simulink model "trajectory_planner"  (R2014b)
settings: Solver=ode45  SolverMode=SingleTasking  StartTime=0.0  StopTime=simtime  RelTol=1e-3
values from neighbouring files (symbols this model uses):
  amax = 255    [workshopB.m]
  amin = -amax    (= -255)    [workshopB.m]
  F_c = 1.5e-3    (= 0.0015)    [workshopB.m]
  J1 = 0.0006    [workshopB.m]
  motor = motor_pars    [workshopB.m]
  n = 5    [workshopB.m]
  t1 = sqrt(rs/amax)    [workshopB.m]
  t2 = t1    [workshopB.m]
  t3 = t1+t2    [workshopB.m]
  Ts = 0.01    [workshopB.m]
libraries: simulink x3
settings Model: Creator=Gabriel  LastModifiedBy=es2lab2
settings SolverCC: ZeroCrossAlgorithm=Adaptive
settings OptimizationCC: BlockReduction=off  BooleanDataType=off  UseDivisionForNetSlopeComputation=off  SimCompilerOptimization=off
settings DebuggingCC: SaveWithParameterizedLinksMsg=none  UnderspecifiedInitializationDetection=Classic  MergeDetectMultiDrivingBlocksExec=none  SignalResolutionControl=TryResolveAllWithWarning  SolverPrmCheckMsg=none  FrameProcessingCompatibilityMsg=error  AllowSymbolicDim=off
settings HardwareCC: TargetUnknown=on
settings RTWCC: RTWCompilerOptimization=off
settings ConfigComp: CovMetricSettings=dw  CovHtmlReporting=on  CovSaveCumulativeToWorkspaceVar=on  CovSaveSingleToWorkspaceVar=on  CovModelRefEnable=Off  CovExternalEMLEnable=off  CovSFcnEnable=off

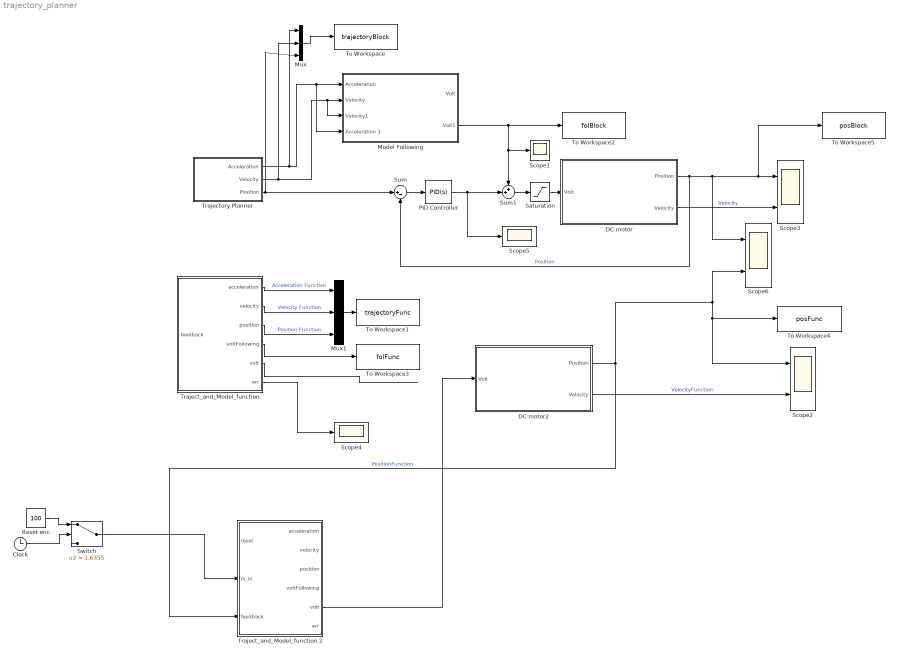
== system trajectory_planner ==
  Clock : Clock
  DC motor : Subsystem
  DC motor2 : Subsystem
  Model Following : Subsystem
  Mux : Mux  Inputs=3
  Mux1 : Mux  Inputs=3
  PID Controller : simulink/Continuous/PID Controller  Controller=PID  TimeDomain=Continuous-time  SampleTime=-1  IntegratorMethod=Forward Euler  FilterMethod=Forward Euler  Form=Parallel  P=1  I=1  D=0  N=100  InitialConditionSource=internal  InitialConditionForIntegrator=0  InitialConditionForFilter=0  ExternalReset=none  LimitOutput=off  UpperSaturationLimit=inf  LowerSaturationLimit=-inf  LinearizeAsGain=on  AntiWindupMode=none  Kb=1  TrackingMode=off  Kt=1  PParamMin=[]  PParamMax=[]  IParamMin=[]  IParamMax=[]  DParamMin=[]  DParamMax=[]  NParamMin=[]  NParamMax=[]  KbParamMin=[]  KbParamMax=[]  KtParamMin=[]  KtParamMax=[]  POutMin=[]  POutMax=[]  IOutMin=[]  IOutMax=[]  DOutMin=[]  DOutMax=[]  NOutMin=[]  NOutMax=[]  KbOutMin=[]  KbOutMax=[]  KtOutMin=[]  KtOutMax=[]  IntegratorOutMin=[]  IntegratorOutMax=[]  FilterOutMin=[]  FilterOutMax=[]  SumOutMin=[]  SumOutMax=[]  SumI1OutMin=[]  SumI1OutMax=[]  SumI2OutMin=[]  SumI2OutMax=[]  SumI3OutMin=[]  SumI3OutMax=[]  SumDOutMin=[]  SumDOutMax=[]  SaturationOutMin=[]  SaturationOutMax=[]  IntegratorContinuousStateAttributes=''  IntegratorStateMustResolveToSignalObject=off  IntegratorRTWStateStorageClass=Auto  FilterContinuousStateAttributes=''  FilterStateMustResolveToSignalObject=off  FilterRTWStateStorageClass=Auto  DifferentiatorICPrevScaledInput=0  DifferentiatorOutMin=[]  DifferentiatorOutMax=[]  UseFilter=on
  Reset enc : Constant  Value=100
  Saturation : Saturate  UpperLimit=24  LowerLimit=-24
  Scope1 : Scope
      settings: TimeRange=7.551351351351352  YMin=-14.3868  YMax=28.08299  SaveName=ScopeData2
  Scope2 : Scope  NumInputPorts=2
      settings: ShowLegends=on  TimeRange=7.551351351351352  YMin=-6.917~-5  YMax=57.3125~5
  Scope3 : Scope  NumInputPorts=2
      settings: ShowLegends=on  TimeRange=7.551351351351352  YMin=-19.9609  YMax=179.64809  SaveName=ScopeData5
  Scope4 : Scope
      settings: TimeRange=7.551351351351352  YMin=-110.7141  YMax=44.80519
  Scope5 : Scope
      settings: TimeRange=7.551351351351352  YMin=-0.000000000000008  YMax=0.000000000000029  SaveName=ScopeData8
  Scope6 : Scope  NumInputPorts=2
      settings: ShowLegends=on  TimeRange=7.551351351351352  YMin=-12.6475~-5  YMax=113.827~5  SaveName=ScopeData3
  Sum : Sum  Inputs=|+-
  Sum1 : Sum  Inputs=++|
  Switch : Switch  Criteria=u2 > Threshold  Threshold=1.6355
  To Workspace : ToWorkspace  VariableName=trajectoryBlock  SaveFormat=Timeseries  SampleTime=-1
  To Workspace1 : ToWorkspace  VariableName=trajectoryFunc  SaveFormat=Timeseries  SampleTime=-1
  To Workspace2 : ToWorkspace  VariableName=folBlock  SaveFormat=Timeseries  SampleTime=-1
  To Workspace3 : ToWorkspace  VariableName=folFunc  SaveFormat=Timeseries  SampleTime=-1
  To Workspace4 : ToWorkspace  VariableName=posFunc  SaveFormat=Timeseries  SampleTime=-1
  To Workspace5 : ToWorkspace  VariableName=posBlock  SaveFormat=Timeseries  SampleTime=-1
  "Traject_and_Model_function " : MATLAB Function  TreatAsAtomicUnit=on  SystemSampleTime=Ts
  Traject_and_Model_function 2 : MATLAB Function  TreatAsAtomicUnit=on  SystemSampleTime=Ts
  Trajectory Planner : Subsystem
  wires:
  Sum/1 -> PID Controller/1
  DC motor/1(Position) -> Sum/2, Scope6/1, To Workspace5/1, Scope3/1  "Position"
  PID Controller/1 -> Sum1/2, Scope5/1
  Trajectory Planner/3(Position) -> Sum/1, Mux/3
  Trajectory Planner/1(Acceleration) -> Mux/1, Model Following/4(Acceleration 1), Model Following/1("Acceleration ")
  Trajectory Planner/2(Velocity) -> Model Following/3(Velocity1), Model Following/2(Velocity), Mux/2
  DC motor/2(Velocity) -> Scope3/2  "Velocity"
  Sum1/1 -> Saturation/1
  Saturation/1 -> DC motor/1(Volt)
  "Traject_and_Model_function "/5(volt) -> ?
  DC motor2/1(Position) -> Traject_and_Model_function 2/3(feedback), Scope6/2, Scope2/1, To Workspace4/1  "PositionFunction"
  DC motor2/2(Velocity) -> Scope2/2  "VelocityFunction"
  Model Following/2(Volt1) -> Sum1/1, Scope1/1, To Workspace2/1
  "Traject_and_Model_function "/1(acceleration) -> Mux1/1  "Acceleration Function"
  "Traject_and_Model_function "/2(velocity) -> Mux1/2  "Velocity Function"
  "Traject_and_Model_function "/3(position) -> Mux1/3  "Position Function"
  Mux/1 -> To Workspace/1
  Mux1/1 -> To Workspace1/1
  "Traject_and_Model_function "/4(voltFollowing) -> To Workspace3/1
  "Traject_and_Model_function "/6(err) -> Scope4/1
  Traject_and_Model_function 2/5(volt) -> DC motor2/1(Volt)
  Reset enc/1 -> Switch/1
  Clock/1 -> Switch/2
  Switch/1 -> Traject_and_Model_function 2/2(rs_in)

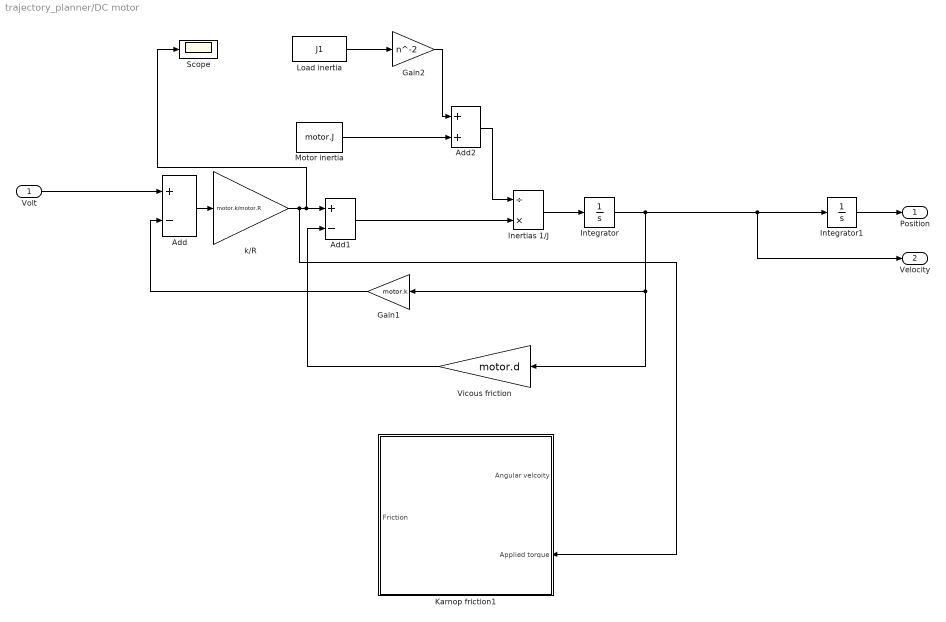
== system trajectory_planner/DC motor ==
  Volt : Inport
  Add : Sum  Inputs=+-
  Add1 : Sum  Inputs=+-
  Add2 : Sum
  Gain1 : Gain  Gain=motor.k
  Gain2 : Gain  Gain=n^-2
  Inertias 1/J : Product  Inputs=/*
  Integrator : Integrator
  Integrator1 : Integrator
  Karnop friction1 : Subsystem
  Load inertia : Constant  Value=J1
  Motor inertia : Constant  Value=motor.J
  Scope : Scope
  Vicous friction : Gain  Gain=motor.d
  "k/R " : Gain  Gain=motor.k/motor.R
  Position : Outport
  Velocity : Outport  Port=2
  wires:
  Vicous friction/1 -> Add1/2
  Add2/1 -> Inertias 1/J/1
  Gain2/1 -> Add2/1
  Load inertia/1 -> Gain2/1
  Motor inertia/1 -> Add2/2
  Integrator/1 -> Integrator1/1, Velocity/1, Vicous friction/1, Gain1/1
  Volt/1 -> Add/1
  Add1/1 -> Inertias 1/J/2
  Integrator1/1 -> Position/1
  Inertias 1/J/1 -> Integrator/1
  "k/R "/1 -> Scope/1, Add1/1, Karnop friction1/2(Applied torque)
  Add/1 -> "k/R "/1
  Gain1/1 -> Add/2

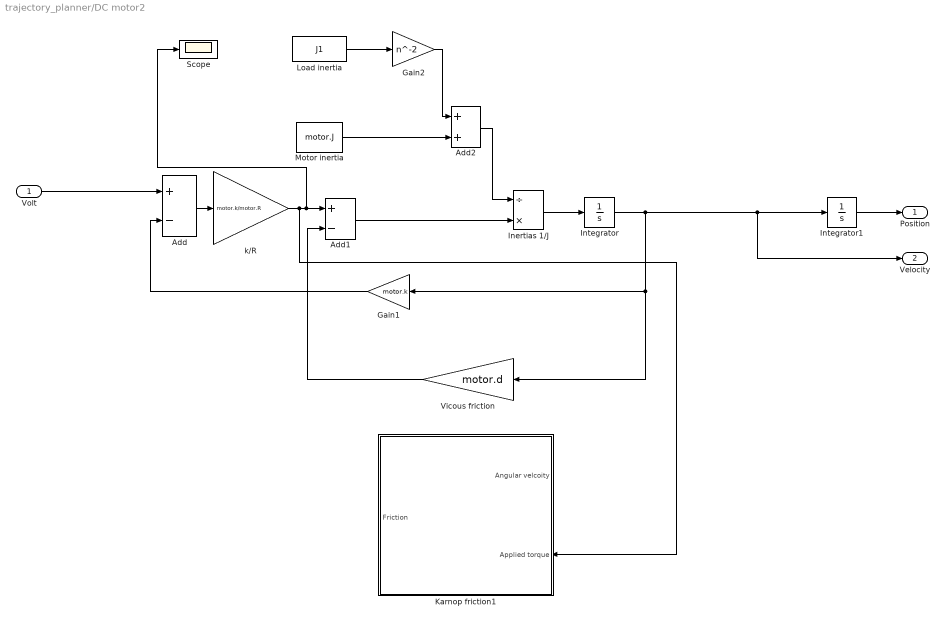
== system trajectory_planner/DC motor2 ==
  Volt : Inport
  Add : Sum  Inputs=+-
  Add1 : Sum  Inputs=+-
  Add2 : Sum
  Gain1 : Gain  Gain=motor.k
  Gain2 : Gain  Gain=n^-2
  Inertias 1/J : Product  Inputs=/*
  Integrator : Integrator
  Integrator1 : Integrator
  Karnop friction1 : Subsystem
  Load inertia : Constant  Value=J1
  Motor inertia : Constant  Value=motor.J
  Scope : Scope
  Vicous friction : Gain  Gain=motor.d
  "k/R " : Gain  Gain=motor.k/motor.R
  Position : Outport
  Velocity : Outport  Port=2
  wires:
  Gain1/1 -> Add/2
  Add/1 -> "k/R "/1
  "k/R "/1 -> Karnop friction1/2(Applied torque), Add1/1, Scope/1
  Inertias 1/J/1 -> Integrator/1
  Integrator1/1 -> Position/1
  Add1/1 -> Inertias 1/J/2
  Volt/1 -> Add/1
  Integrator/1 -> Vicous friction/1, Gain1/1, Velocity/1, Integrator1/1
  Motor inertia/1 -> Add2/2
  Load inertia/1 -> Gain2/1
  Gain2/1 -> Add2/1
  Add2/1 -> Inertias 1/J/1
  Vicous friction/1 -> Add1/2

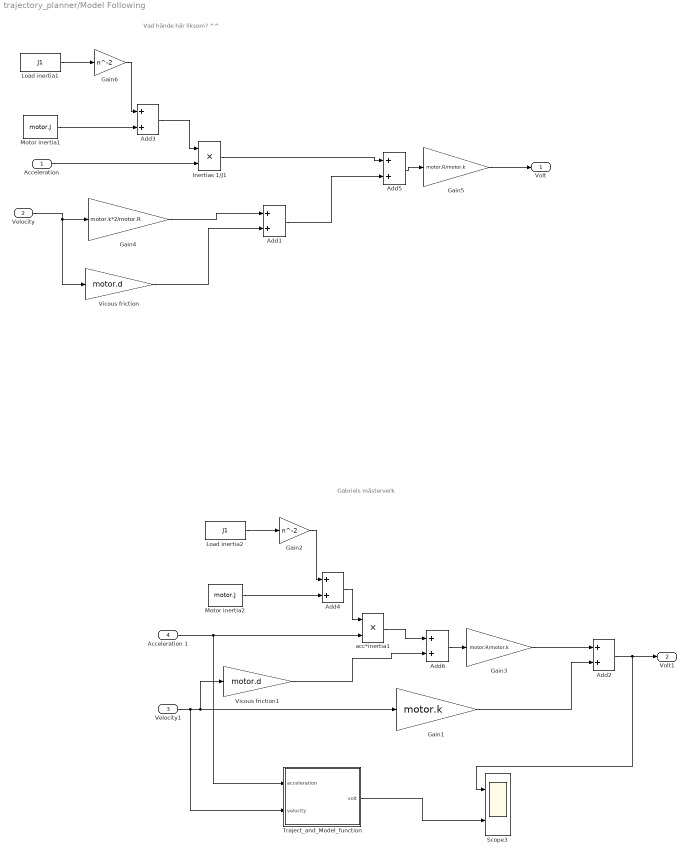
== system trajectory_planner/Model Following ==
  note: Vad hände här liksom? ^^
  note: Gabriels mästerverk
  "Acceleration " : Inport
  Velocity : Inport  Port=2
  Velocity1 : Inport  Port=3
  Acceleration 1 : Inport  Port=4
  Add{1..6} (6 alike) : Sum
  Gain1 : Gain  Gain=motor.k
  Gain2 : Gain  Gain=n^-2
  Gain3 : Gain  Gain=motor.R/motor.k
  Gain4 : Gain  Gain=motor.k*2/motor.R
  Gain5 : Gain  Gain=motor.R/motor.k
  Gain6 : Gain  Gain=n^-2
  Inertias 1/J1 : Product  Inputs=**
  Load inertia1 : Constant  Value=J1
  Load inertia2 : Constant  Value=J1
  Motor inertia1 : Constant  Value=motor.J
  Motor inertia2 : Constant  Value=motor.J
  Scope3 : Scope  NumInputPorts=2
      settings: ShowLegends=on  TimeRange=7.551351351351352  YMin=-14.3868  YMax=28.08299  SaveName=ScopeData4
  "Traject_and_Model_function " : MATLAB Function  TreatAsAtomicUnit=on  SystemSampleTime=Ts
  Vicous friction : Gain  Gain=motor.d
  Vicous friction1 : Gain  Gain=motor.d
  acc*inertia1 : Product  Inputs=**
  Volt : Outport
  Volt1 : Outport  Port=2
  wires:
  "Acceleration "/1 -> Inertias 1/J1/2
  Velocity/1 -> Vicous friction/1, Gain4/1
  Add3/1 -> Inertias 1/J1/1
  Gain6/1 -> Add3/1
  Load inertia1/1 -> Gain6/1
  Motor inertia1/1 -> Add3/2
  Vicous friction/1 -> Add1/2
  Gain5/1 -> Volt/1
  Add5/1 -> Gain5/1
  Inertias 1/J1/1 -> Add5/1
  Gain4/1 -> Add1/1
  Add1/1 -> Add5/2
  Velocity1/1 -> "Traject_and_Model_function "/2(velocity), Gain1/1, Vicous friction1/1
  Gain1/1 -> Add2/2
  Acceleration 1/1 -> "Traject_and_Model_function "/1(acceleration), acc*inertia1/2
  Add4/1 -> acc*inertia1/1
  Gain2/1 -> Add4/1
  Load inertia2/1 -> Gain2/1
  Motor inertia2/1 -> Add4/2
  Vicous friction1/1 -> Add6/2
  acc*inertia1/1 -> Add6/1
  Add6/1 -> Gain3/1
  Gain3/1 -> Add2/1
  Add2/1 -> Scope3/1, Volt1/1
  "Traject_and_Model_function "/1(volt) -> Scope3/2

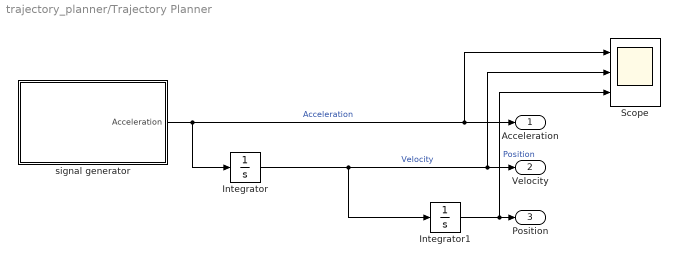
== system trajectory_planner/Trajectory Planner ==
  Integrator : Integrator
  Integrator1 : Integrator
  Scope : Scope  NumInputPorts=3
      settings: ShowLegends=on  YMin=-318.75~-5~-5  YMax=318.75~5~5
  signal generator : Subsystem
  Acceleration : Outport
  Velocity : Outport  Port=2
  Position : Outport  Port=3
  wires:
  signal generator/1(Acceleration) -> Integrator/1, Scope/1, Acceleration/1  "Acceleration"
  Integrator/1 -> Scope/2, Velocity/1, Integrator1/1  "Velocity"
  Integrator1/1 -> Scope/3, Position/1  "Position"

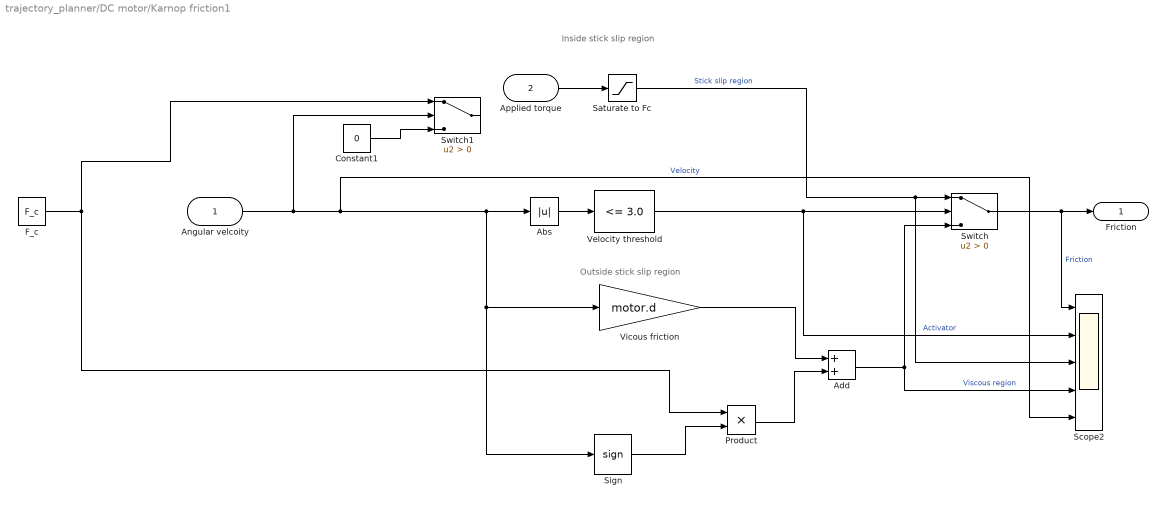
== system trajectory_planner/DC motor/Karnop friction1 ==
  note: Outside stick slip region
  note: Inside stick slip region
  Angular velcoity : Inport
  Applied torque : Inport  Port=2
  Abs : Abs  ZeroCross=off
  Add : Sum
  Constant1 : Constant  Value=0
  F_c : Constant  Value=F_c
  Product : Product
  Saturate to Fc : Saturate  UpperLimit=F_c  LowerLimit=-F_c  ZeroCross=off
  Scope2 : Scope  NumInputPorts=5
  Sign : Signum  ZeroCross=off
  Switch : Switch  Criteria=u2 > Threshold  ZeroCross=off
  Switch1 : Switch  Criteria=u2 > Threshold  ZeroCross=off
  "Velocity threshold " : simulink/Logic and Bit Operations/Compare To Constant  relop=<=  const=3.0  OutDataTypeStr=boolean
  Vicous friction : Gain  Gain=motor.d
  Friction : Outport
  wires:
  Applied torque/1 -> Saturate to Fc/1
  Add/1 -> Scope2/4, Switch/3  "Viscous region"
  Sign/1 -> Product/2
  F_c/1 -> Product/1, Switch1/1
  Vicous friction/1 -> Add/1
  Product/1 -> Add/2
  Abs/1 -> "Velocity threshold "/1
  "Velocity threshold "/1 -> Switch/2, Scope2/2  "Activator"
  Angular velcoity/1 -> Switch1/2, Sign/1, Vicous friction/1, Abs/1, Scope2/5  "Velocity"
  Switch/1 -> Friction/1, Scope2/1  "Friction"
  Saturate to Fc/1 -> Switch/1, Scope2/3  "Stick slip region"
  Constant1/1 -> Switch1/3

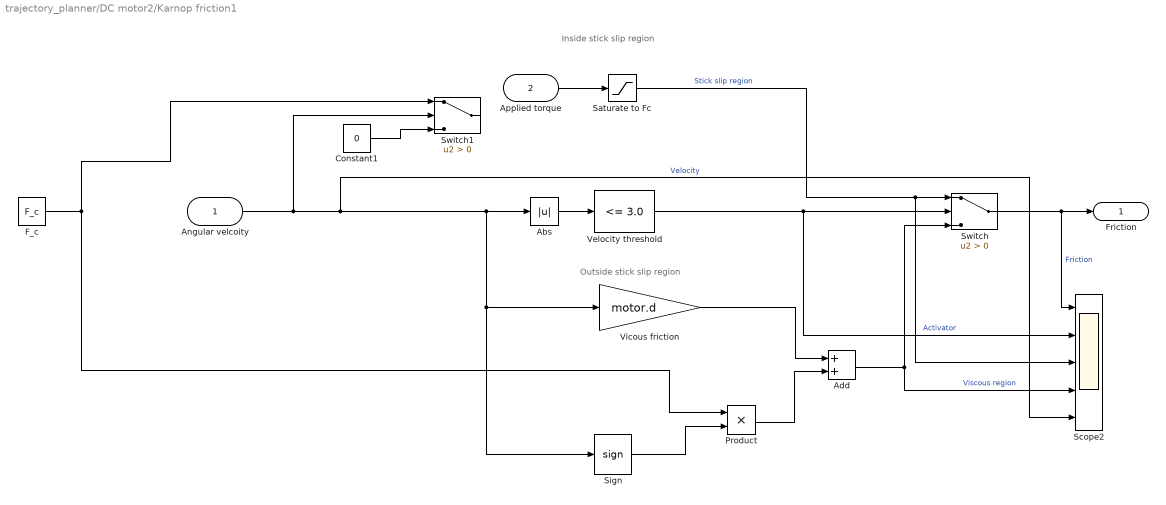
== system trajectory_planner/DC motor2/Karnop friction1 ==
  note: Inside stick slip region
  note: Outside stick slip region
  Angular velcoity : Inport
  Applied torque : Inport  Port=2
  Abs : Abs  ZeroCross=off
  Add : Sum
  Constant1 : Constant  Value=0
  F_c : Constant  Value=F_c
  Product : Product
  Saturate to Fc : Saturate  UpperLimit=F_c  LowerLimit=-F_c  ZeroCross=off
  Scope2 : Scope  NumInputPorts=5
  Sign : Signum  ZeroCross=off
  Switch : Switch  Criteria=u2 > Threshold  ZeroCross=off
  Switch1 : Switch  Criteria=u2 > Threshold  ZeroCross=off
  "Velocity threshold " : simulink/Logic and Bit Operations/Compare To Constant  relop=<=  const=3.0  OutDataTypeStr=boolean
  Vicous friction : Gain  Gain=motor.d
  Friction : Outport
  wires:
  Constant1/1 -> Switch1/3
  Saturate to Fc/1 -> Scope2/3, Switch/1  "Stick slip region"
  Switch/1 -> Scope2/1, Friction/1  "Friction"
  Angular velcoity/1 -> Scope2/5, Abs/1, Vicous friction/1, Sign/1, Switch1/2  "Velocity"
  "Velocity threshold "/1 -> Scope2/2, Switch/2  "Activator"
  Abs/1 -> "Velocity threshold "/1
  Product/1 -> Add/2
  Vicous friction/1 -> Add/1
  F_c/1 -> Switch1/1, Product/1
  Sign/1 -> Product/2
  Add/1 -> Switch/3, Scope2/4  "Viscous region"
  Applied torque/1 -> Saturate to Fc/1

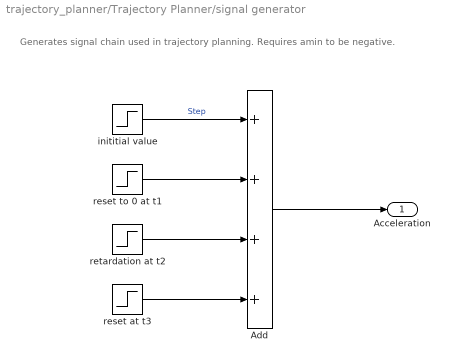
== system trajectory_planner/Trajectory Planner/signal generator ==
  note: Generates signal chain used in trajectory planning. Requires amin to be negative.
  Add : Sum  Inputs=++++
  "inititial value " : Step  Time=0  After=amax  SampleTime=0
  reset at t3 : Step  Time=t3  After=-amin  SampleTime=0
  reset to 0 at t1 : Step  Time=t1  After=-amax  SampleTime=0
  retardation at t2 : Step  Time=t2  After=amin  SampleTime=0
  Acceleration : Outport
  wires:
  reset at t3/1 -> Add/4
  Add/1 -> Acceleration/1
  retardation at t2/1 -> Add/3
  "inititial value "/1 -> Add/1  "Step"
  reset to 0 at t1/1 -> Add/2

== matlab function trajectory_planner/Model Following/Traject_and_Model_function  ==
  data: volt output; acceleration input; velocity input
function volt   = Controller(acceleration,velocity)
%#codegen

%% MODEL FOLLOWING PART

% Model Following variables
J1 = 6e-4;
motor_j = 7.46e-7;
n = 5;
motor_k = 0.0697;
motor_R = 112;
motor_d = 1e-5;
%% Input Acceleration Part

accPart = acceleration*(J1/(n^2)+motor_j);
 
%% Input Velocity Part
 
velPartK = velocity*motor_k;
velPartD = velocity*motor_d;
 
%%Output
 
volt = (accPart+velPartD)*motor_R/motor_k + velPartK;


end

== matlab function trajectory_planner/Traject_and_Model_function 2 ==
  data: reset input; rs_in input; acceleration output; velocity output; position output; voltFollowing output; volt output; feedback input; err output
function [acceleration,velocity,position,voltFollowing,volt,err]  = Controller(reset,rs_in,feedback)
%#codegen
% PERSISTENT VARIABLES
persistent time;
if isempty(time)
    time = 0;
end

persistent oldAcc;
if isempty(oldAcc)
    oldAcc = 0;
end

persistent oldVel;
if isempty(oldVel)
    oldVel = 0;
end

persistent oldPos;
if isempty(oldPos)
    oldPos = 0;
end
persistent rs;
if isempty(rs)
    rs = 0;
end
%Update "time"

if(reset == 1)
    position = 0;
    velocity = 0;
    acceleration = 0;
    time = 0;
end
if(rs_in ~= rs)
    position = 0;
    velocity = 0;
    acceleration = 0;
    time = 0;
end
rs = rs_in;

% Trajectory Planner Variables
Ts = 0.01;
vmax = 270;% 252;
amax = 255; %369;
amin = -amax;
t1 = sqrt(rs/amax);
t2 = t1;
t3 = t1+t2;
voltmax = 24;

%Initial Value block
out1 = amax;
%%SIGNAL GENERATOR
%Reset to 0 at t1 block
out2 = 0;
if(time >= t1)
    out2 = amin;
end

%retardation at t2 block
out3 = 0;
if(time >= t2)
    out3 = amin;
end

% Reset at t3 block
out4 = 0;
if(time >= t3)
    out4 = amax;
end

acceleration = out1+out2+out3+out4;
oldAcc = acceleration;
%% INTEGRATOR PARTS
%For velocity
velocity = oldVel + Ts*(acceleration+oldAcc)/2;
oldVel = velocity;

%For position
position = oldPos + Ts*(velocity+oldVel)/2;

oldPos = position;

%% MODEL FOLLOWING PART

% Model Following variables
J1 = 0.0006;
motor_j = 7.46e-7;
n = 5;
motor_k = 0.0697;
motor_R = 112;
motor_d = 1e-5;
%% Input Acceleration Part

accPart = acceleration*(J1/(n^2)+motor_j);
 
%% Input Velocity Part
 
velPartK = velocity*motor_k;
velPartD = velocity*motor_d;
 
%%Output
 
voltFollowing = (accPart+velPartD)*motor_R/motor_k + velPartK;


%% PID CONTROLLER

% PERSISTENT VARIABLES
persistent oldErr
if isempty(oldErr)
    oldErr = 0;
end
persistent olderErr
if isempty(olderErr)
    olderErr=0;
end
persistent oldPIDVolt
if isempty(oldPIDVolt)
    oldPIDVolt = 0;
end
persistent olderPIDVolt
if isempty(olderPIDVolt)
    olderPIDVolt = 0;
end
% PID parameters
s2 = 1348;
s1 = -1899;
s0 = 692;
r0 = 0.89;

% Error
err = position - feedback;

%%PID
PIDVolt = s2*err+s1*oldErr+s0*olderErr+r0*olderPIDVolt-(r0-1)*oldPIDVolt;
olderPIDVolt = oldPIDVolt;
oldPIDVolt = PIDVolt;
olderErr = oldErr;
oldErr = err;
%% OUTPUT

volt = voltFollowing+PIDVolt;

if(volt >= voltmax)
    volt = voltmax;
elseif(volt <= -voltmax)
    volt = -voltmax;
end


time = time +Ts;

end

== matlab function trajectory_planner/Traject_and_Model_function  ==
  data: acceleration output; velocity output; position output; voltFollowing output; volt output; feedback input; err output
function [acceleration,velocity,position,voltFollowing,volt,err]  = Controller(feedback)
%#codegen
% PERSISTENT VARIABLES
persistent time;
if isempty(time)
    time = 0;
end

persistent oldAcc;
if isempty(oldAcc)
    oldAcc = 0;
end

persistent oldVel;
if isempty(oldVel)
    oldVel = 0;
end

persistent oldPos;
if isempty(oldPos)
    oldPos = 0;
end
%Update "time"


% Trajectory Planner Variables
Ts = 0.01;
vmax = 270;% 252;
amax = 255; %369;
amin = -amax;
rs = 100;
t1 = sqrt(rs/amax);
t2 = t1;
t3 = t1+t2;
voltmax = 24;

%Initial Value block
out1 = amax;
%%SIGNAL GENERATOR
%Reset to 0 at t1 block
out2 = 0;
if(time >= t1)
    out2 = amin;
end

%retardation at t2 block
out3 = 0;
if(time >= t2)
    out3 = amin;
end

% Reset at t3 block
out4 = 0;
if(time >= t3)
    out4 = amax;
end

acceleration = out1+out2+out3+out4;
oldAcc = acceleration;
%% INTEGRATOR PARTS
%For velocity
velocity = oldVel + Ts*(acceleration+oldAcc)/2;
oldVel = velocity;

%For position
position = oldPos + Ts*(velocity+oldVel)/2;

oldPos = position;

%% MODEL FOLLOWING PART

% Model Following variables
J1 = 6e-4;
motor_j = 7.46e-7;
n = 5;
motor_k = 0.0697;
motor_R = 112;
motor_d = 1e-5;
%% Input Acceleration Part

accPart = acceleration*(J1/(n^2)+motor_j);
 
%% Input Velocity Part
 
velPartK = velocity*motor_k;
velPartD = velocity*motor_d;
 
%%Output
 
voltFollowing = (accPart+velPartD)*motor_R/motor_k + velPartK;


%% PID CONTROLLER

% PERSISTENT VARIABLES
persistent oldErr
if isempty(oldErr)
    oldErr = 0;
end
persistent olderErr
if isempty(olderErr)
    olderErr=0;
end
persistent oldPIDVolt
if isempty(oldPIDVolt)
    oldPIDVolt = 0;
end
persistent olderPIDVolt
if isempty(olderPIDVolt)
    olderPIDVolt = 0;
end
% PID parameters
s2 = 1348;
s1 = -1899;
s0 = 692;
r0 = 0.89;

% Error
err = position - feedback;

%%PID
PIDVolt = s2*err+s1*oldErr+s0*olderErr+r0*olderPIDVolt-(r0-1)*oldPIDVolt;
olderPIDVolt = oldPIDVolt;
oldPIDVolt = PIDVolt;
olderErr = oldErr;
oldErr = err;
%% OUTPUT

volt = voltFollowing+PIDVolt;

if(volt >= voltmax)
    volt = voltmax;
elseif(volt <= -voltmax)
    volt = -voltmax;
end


time = time +Ts;

end
